simulink model "whole"  (R2014a)
settings: Solver=ode45  StartTime=0.0  StopTime=20  RelTol=1e-3
libraries: simulink_extras x2, simulink x1
settings Model: Creator=Administrator  LastModifiedBy=Administrator

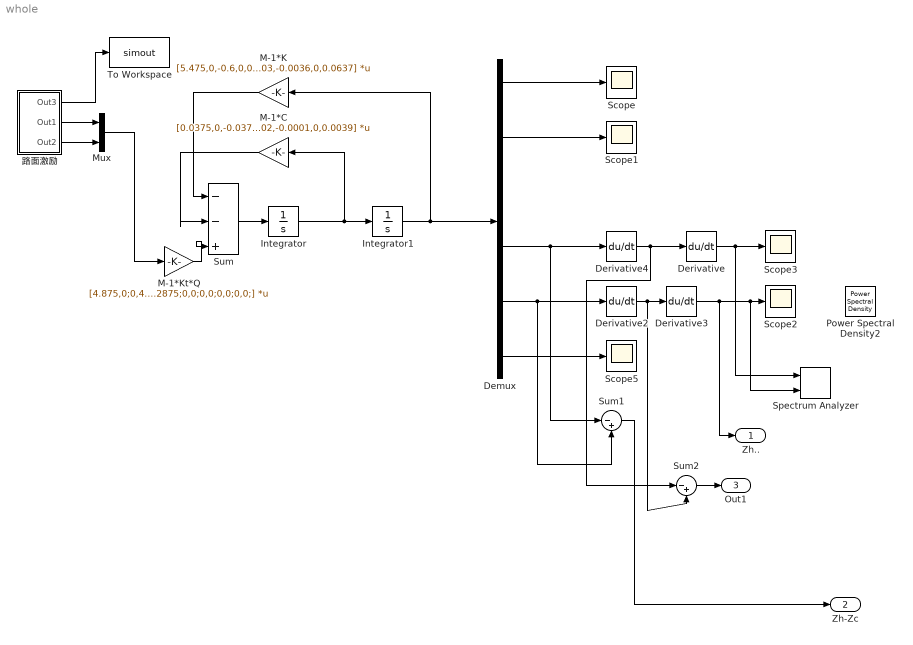
== system whole ==
  Demux : Demux  Outputs=6
  Derivative{,2..4} (4 alike) : Derivative
  Integrator : Integrator
  Integrator1 : Integrator
  M-1*C : Gain  Gain=[0.0375,0,-0.0375,0,0,0.0506;0,0.033,-0.033,0,0,-0.0379;-0.0022,-0.0022,0.0046,-0.0002,0,-0.0003;0,0,-0.0021,0.0043,-0.0021,-0.0012;0,0,0,-0.0135,0.0135,0;0.0017,-0.0014,-0.0002,-0.0001,0,0.0039]  Multiplication=Matrix(K*u)
  M-1*K : Gain  Gain=[5.475,0,-0.6,0,0,0.81;0,4.8132,-0.5275,0,0,-0.6066;-0.0348,-0.0348,0.0812,0.0116,0,-0.0006;0,0,0.1143,0.1714,-0.0571,-0.0629;0,0,0,-0.3604,0.3604,0;0.0265,-0.0226,-0.0003,-0.0036,0,0.0637]  Multiplication=Matrix(K*u)
  M-1*Kt*Q : Gain  Gain=[4.875,0;0,4.2875;0,0;0,0;0,0;0,0;]  Multiplication=Matrix(K*u)
  Mux : Mux  Inputs=2
  Power Spectral Density2 : simulink_extras/Additional Sinks/Power Spectral Density  npts=128  fftpts=512  HowOften=64  sampleT=0.1
  Scope{,1..3,5} (5 alike) : Scope
      Scope2 settings: SaveName=ScopeData2
      Scope3 settings: SaveName=ScopeData3
      Scope5 settings: SaveName=ScopeData5
  Spectrum Analyzer : simulink_extras/Additional Sinks/Spectrum Analyzer  npts=256  fftpts=256  HowOften=64  sampleT=0.1
  Sum : Sum  Inputs=|--+
  Sum1 : Sum  Inputs=|-+
  Sum2 : Sum  Inputs=|-+
  To Workspace : ToWorkspace  VariableName=simout  SaveFormat=Structure With Time  SampleTime=-1
  "路面激励 " : Subsystem
  Zh.. : Outport
  Zh-Zc : Outport  Port=2
  Out1 : Outport  Port=3
  wires:
  "路面激励 "/1(Out3) -> To Workspace/1
  Sum/1 -> Integrator/1
  M-1*Kt*Q/1 -> Sum/3
  Integrator1/1 -> M-1*K/1, Demux/1
  M-1*K/1 -> Sum/1
  Integrator/1 -> M-1*C/1, Integrator1/1
  M-1*C/1 -> Sum/2
  Demux/1 -> Scope/1
  Demux/2 -> Scope1/1
  Demux/6 -> Scope5/1
  Demux/5 -> Sum1/2, Derivative2/1
  Demux/4 -> Sum1/1, Derivative4/1
  "路面激励 "/2(Out1) -> Mux/1
  "路面激励 "/3(Out2) -> Mux/2
  Derivative2/1 -> Sum2/2, Derivative3/1
  Derivative3/1 -> Spectrum Analyzer/2, Scope2/1, Zh../1
  Derivative4/1 -> Derivative/1, Sum2/1
  Mux/1 -> M-1*Kt*Q/1
  Sum2/1 -> Out1/1
  Sum1/1 -> Zh-Zc/1
  Derivative/1 -> Spectrum Analyzer/1, Scope3/1

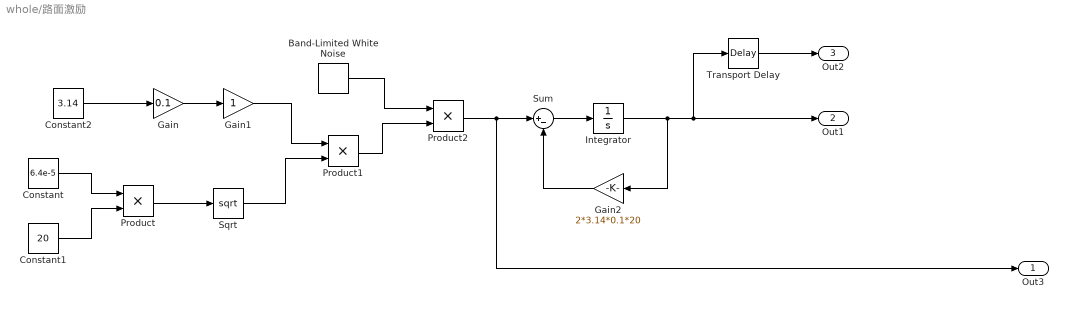
== system whole/路面激励  ==
  Band-Limited White Noise : simulink/Sources/Band-Limited White Noise  Cov=[0.1]  Ts=0.1  seed=[23341]
  Constant : Constant  Value=6.4e-5
  Constant1 : Constant  Value=20
  Constant2 : Constant  Value=3.14
  Gain : Gain  Gain=0.1
  Gain1 : Gain
  Gain2 : Gain  Gain=2*3.14*0.1*20
  Integrator : Integrator
  Product : Product
  Product1 : Product
  Product2 : Product
  Sqrt : Sqrt  SaturateOnIntegerOverflow=on
  Sum : Sum  Inputs=|+-
  Transport Delay : TransportDelay
  Out3 : Outport
  Out1 : Outport  Port=2
  Out2 : Outport  Port=3
  wires:
  Gain2/1 -> Sum/2
  Product/1 -> Sqrt/1
  Gain/1 -> Gain1/1
  Product1/1 -> Product2/2
  Constant/1 -> Product/1
  Sqrt/1 -> Product1/2
  Constant1/1 -> Product/2
  Constant2/1 -> Gain/1
  Band-Limited White Noise/1 -> Product2/1
  Product2/1 -> Out3/1, Sum/1
  Integrator/1 -> Transport Delay/1, Out1/1, Gain2/1
  Sum/1 -> Integrator/1
  Gain1/1 -> Product1/1
  Transport Delay/1 -> Out2/1
